simulink model "Aufiero_slew_pointing"  (R2021a)
settings: Solver=VariableStepAuto  StartTime=0.0  StopTime=100  RelTol=1e-3
settings Model: Creator=691615  LastModifiedBy=aufie
settings SolverCC: ZeroCrossAlgorithm=Adaptive  AlgebraicLoopSolver=TrustRegion
settings DebuggingCC: IgnoredZcDiagnostic=none  SFMachineParentedDataDiag=warning

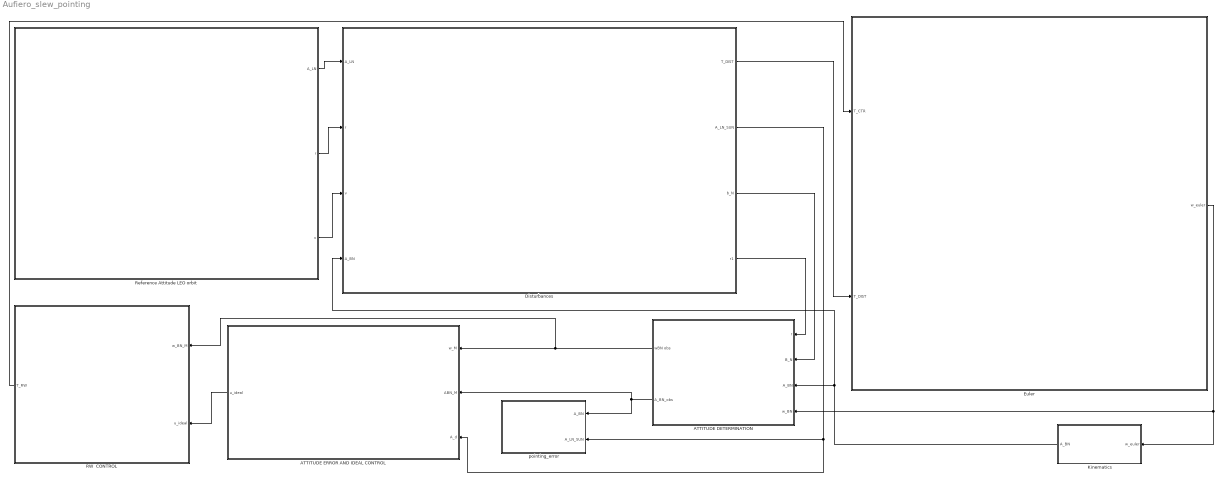
== system Aufiero_slew_pointing ==
  ATTITUDE DETERMINATION : Subsystem
  ATTITUDE ERROR AND IDEAL CONTROL : Subsystem
  Disturbances : Subsystem
  Euler : Subsystem
  Kinematics : Subsystem
  RW  CONTROL : Subsystem
  Reference Attitude LEO orbit : Subsystem
  pointing_error : Subsystem
  wires:
  ATTITUDE ERROR AND IDEAL CONTROL/1(u_ideal) -> RW  CONTROL/2(u_ideal)
  Kinematics/1(A_BN) -> ATTITUDE DETERMINATION/3(A_BN), Disturbances/4(A_BN)
  ATTITUDE DETERMINATION/2(A_BN_obs) -> ATTITUDE ERROR AND IDEAL CONTROL/2(ABN_M), pointing_error/1(A_BN)
  ATTITUDE DETERMINATION/1(wBN obs) -> ATTITUDE ERROR AND IDEAL CONTROL/1(w_M), RW  CONTROL/1(w_BN_M)
  Euler/1(w_euler) -> Kinematics/1(w_euler), ATTITUDE DETERMINATION/4(w_BN)
  RW  CONTROL/1(T_RW) -> Euler/1(T_CTR)
  Reference Attitude LEO orbit/3(v) -> Disturbances/3(v)
  Reference Attitude LEO orbit/1(A_LN) -> Disturbances/1(A_LN)
  Reference Attitude LEO orbit/2(r) -> Disturbances/2(r)
  Disturbances/1(T_DIST) -> Euler/2(T_DIST)
  Disturbances/2(A_LN_SUN) -> ATTITUDE ERROR AND IDEAL CONTROL/3(A_d), pointing_error/2(A_LN_SUN)
  Disturbances/4(r1) -> ATTITUDE DETERMINATION/1(r)
  Disturbances/3(b_N) -> ATTITUDE DETERMINATION/2(B_N)

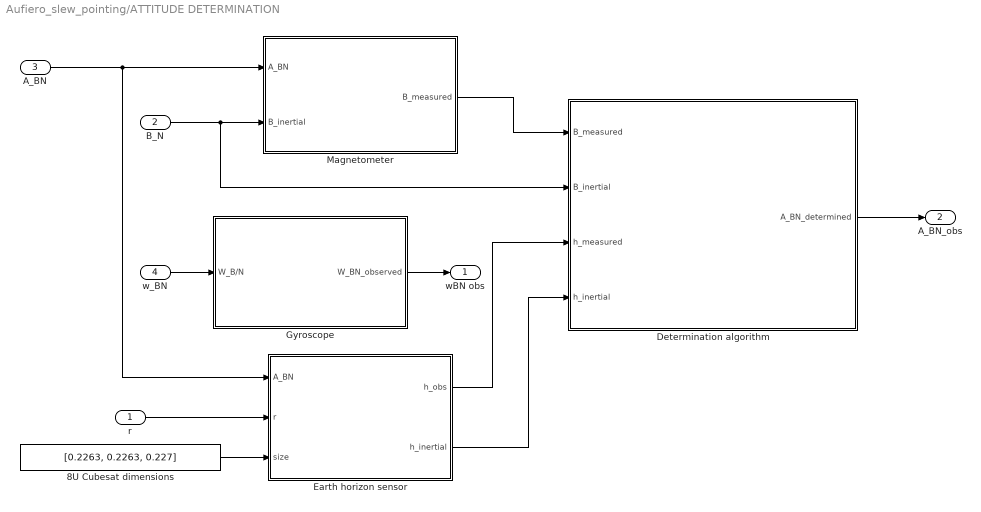
== system Aufiero_slew_pointing/ATTITUDE DETERMINATION ==
  r : Inport
  B_N : Inport  Port=2
  A_BN : Inport  Port=3
  w_BN : Inport  Port=4
  8U Cubesat dimensions : Constant  Value=[0.2263, 0.2263, 0.227]
  "Determination algorithm " : Subsystem
  Earth horizon sensor : Subsystem
  Gyroscope : Subsystem
  Magnetometer : Subsystem
  wBN obs : Outport  VectorParamsAs1DForOutWhenUnconnected=off
  A_BN_obs : Outport  Port=2  VectorParamsAs1DForOutWhenUnconnected=off
  wires:
  Earth horizon sensor/2(h_inertial) -> "Determination algorithm "/4(h_inertial)
  B_N/1 -> "Determination algorithm "/2(B_inertial), Magnetometer/2(B_inertial)
  w_BN/1 -> Gyroscope/1(W_B/N)
  "Determination algorithm "/1(A_BN_determined) -> A_BN_obs/1
  A_BN/1 -> Earth horizon sensor/1(A_BN), Magnetometer/1(A_BN)
  Earth horizon sensor/1(h_obs) -> "Determination algorithm "/3(h_measured)
  r/1 -> Earth horizon sensor/2(r)
  Gyroscope/1(W_BN_observed) -> wBN obs/1
  Magnetometer/1(B_measured) -> "Determination algorithm "/1(B_measured)
  8U Cubesat dimensions/1 -> Earth horizon sensor/3(size)

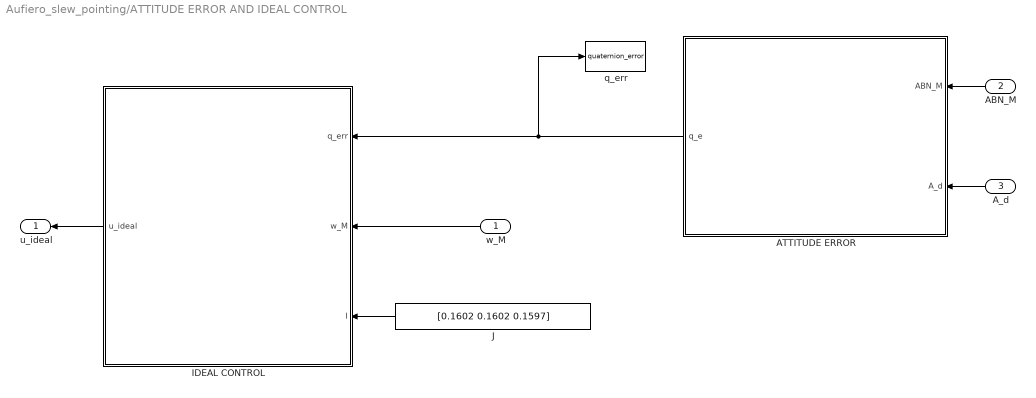
== system Aufiero_slew_pointing/ATTITUDE ERROR AND IDEAL CONTROL ==
  w_M : Inport
  ABN_M : Inport  Port=2
  A_d : Inport  Port=3
  ATTITUDE ERROR : MATLAB Function  TreatAsAtomicUnit=on
  IDEAL CONTROL : MATLAB Function  TreatAsAtomicUnit=on
  J : Constant  Value=[0.1602 0.1602 0.1597]
  q_err : ToWorkspace  VariableName=quaternion_error  SaveFormat=Timeseries  SampleTime=-1
  u_ideal : Outport  VectorParamsAs1DForOutWhenUnconnected=off
  wires:
  J/1 -> IDEAL CONTROL/3(I)
  w_M/1 -> IDEAL CONTROL/2(w_M)
  ABN_M/1 -> ATTITUDE ERROR/1(ABN_M)
  IDEAL CONTROL/1(u_ideal) -> u_ideal/1
  ATTITUDE ERROR/1(q_e) -> q_err/1, IDEAL CONTROL/1(q_err)
  A_d/1 -> ATTITUDE ERROR/2(A_d)

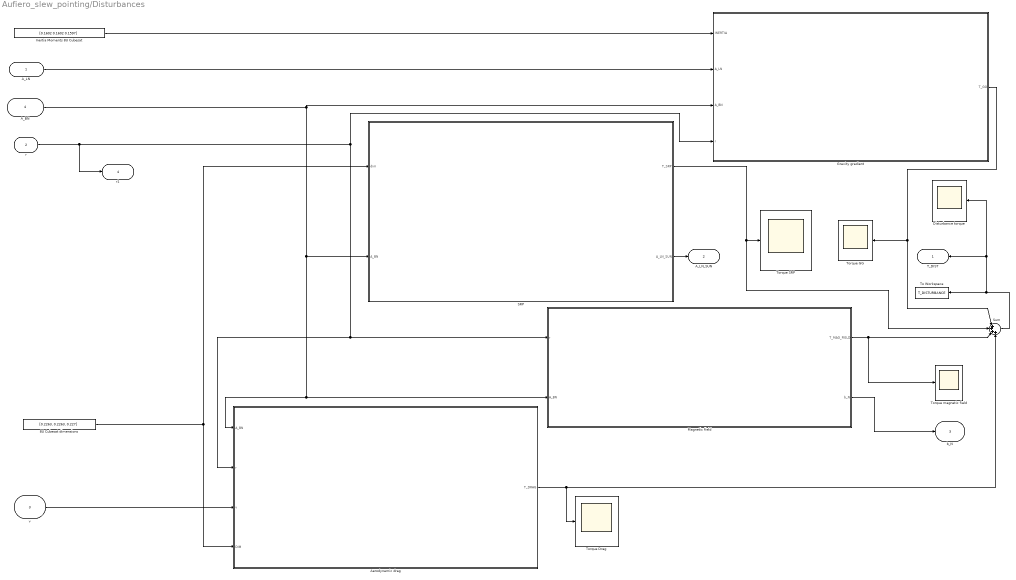
== system Aufiero_slew_pointing/Disturbances ==
  A_LN : Inport
  r : Inport  Port=2
  v : Inport  Port=3
  A_BN : Inport  Port=4
  8U Cubesat dimensions : Constant  Value=[0.2263, 0.2263, 0.227]
  Aerodynamic drag : Subsystem
  Disturbance torque : Scope
  Gravity gradient : Subsystem
  Inertia Moments 8U Cubesat : Constant  Value=[0.1602 0.1602 0.1597]
  Magnetic field : Subsystem
  SRP : Subsystem
  Sum : Sum  Inputs=|++++
  To Workspace : ToWorkspace  VariableName=T_DISTURBANCE  SaveFormat=Timeseries  SampleTime=-1
  Torque Drag : Scope
  Torque GG : Scope
  Torque SRP : Scope
  Torque magnetic field : Scope
  T_DIST : Outport  VectorParamsAs1DForOutWhenUnconnected=off
  A_LN_SUN : Outport  Port=2  VectorParamsAs1DForOutWhenUnconnected=off
  b_N : Outport  Port=3  VectorParamsAs1DForOutWhenUnconnected=off
  r1 : Outport  Port=4  VectorParamsAs1DForOutWhenUnconnected=off
  wires:
  r/1 -> Gravity gradient/4(r), Aerodynamic drag/2(r), Magnetic field/1(r), r1/1
  v/1 -> Aerodynamic drag/3(v)
  8U Cubesat dimensions/1 -> SRP/1(dim), Aerodynamic drag/4(DIM)
  Inertia Moments 8U Cubesat/1 -> Gravity gradient/1(INERTIA)
  A_LN/1 -> Gravity gradient/2(A_LN)
  Gravity gradient/1(T_GG) -> Torque GG/1, Sum/1
  SRP/1(T_SRP) -> Sum/2, Torque SRP/1
  Aerodynamic drag/1(T_DRAG) -> Sum/4, Torque Drag/1
  Magnetic field/1(T_MAG_FIELD) -> Torque magnetic field/1, Sum/3
  Magnetic field/2(b_N) -> b_N/1
  A_BN/1 -> Gravity gradient/3(A_BN), SRP/2(A_BN), Aerodynamic drag/1(A_BN), Magnetic field/2(A_BN)
  Sum/1 -> Disturbance torque/1, T_DIST/1, To Workspace/1
  SRP/2(A_LN_SUN) -> A_LN_SUN/1

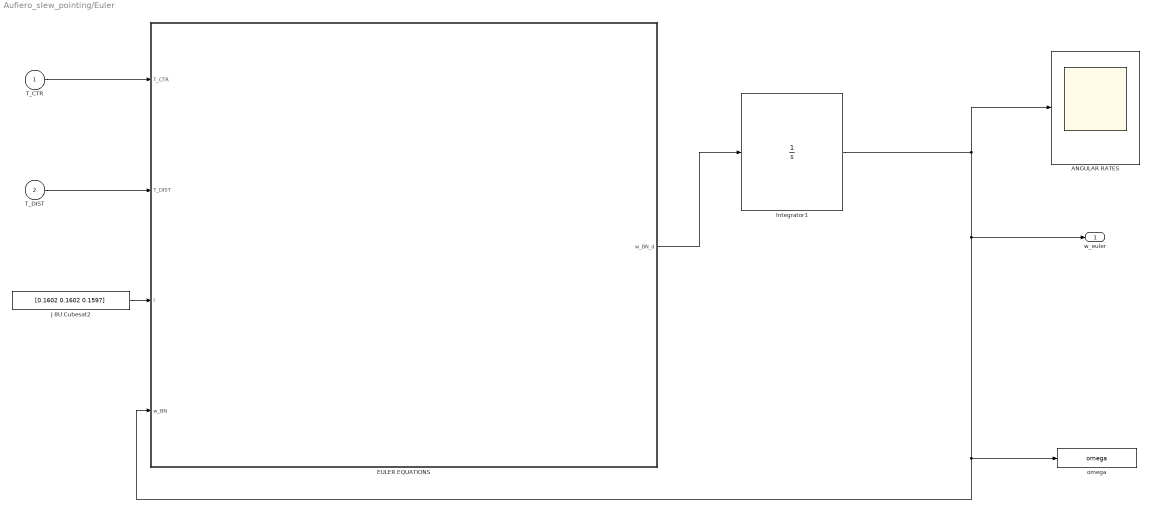
== system Aufiero_slew_pointing/Euler ==
  T_CTR : Inport
  T_DIST : Inport  Port=2
  ANGULAR RATES : Scope
  EULER EQUATIONS : MATLAB Function  TreatAsAtomicUnit=on
  Integrator1 : Integrator  InitialCondition=[0 0 0]
  J 8U Cubesat2 : Constant  Value=[0.1602 0.1602 0.1597]
  omega : ToWorkspace  VariableName=omega  SaveFormat=Timeseries  SampleTime=-1
  w_euler : Outport  VectorParamsAs1DForOutWhenUnconnected=off
  wires:
  T_CTR/1 -> EULER EQUATIONS/1(T_CTR)
  EULER EQUATIONS/1(w_BN_d) -> Integrator1/1
  T_DIST/1 -> EULER EQUATIONS/2(T_DIST)
  Integrator1/1 -> ANGULAR RATES/1, w_euler/1, EULER EQUATIONS/4(w_BN), omega/1
  J 8U Cubesat2/1 -> EULER EQUATIONS/3(I)

== system Aufiero_slew_pointing/Kinematics ==
  w_euler : Inport
  Attitude matrix quaternions : MATLAB Function  TreatAsAtomicUnit=on
  Integrator2 : Integrator  InitialCondition=[0 0 0 1]
  "Orthonorm. quaternions " : MATLAB Function  TreatAsAtomicUnit=on
  "Quaternions kinematics " : MATLAB Function  TreatAsAtomicUnit=on
  A_BN : Outport  VectorParamsAs1DForOutWhenUnconnected=off
  wires:
  w_euler/1 -> "Quaternions kinematics "/1(w)
  "Orthonorm. quaternions "/1(q_ortho) -> Attitude matrix quaternions/1(q), "Quaternions kinematics "/2(q)
  "Quaternions kinematics "/1(q_dot) -> Integrator2/1
  Integrator2/1 -> "Orthonorm. quaternions "/1(q)
  Attitude matrix quaternions/1(A_BN) -> A_BN/1

== system Aufiero_slew_pointing/RW  CONTROL ==
  w_BN_M : Inport
  u_ideal : Inport  Port=2
  RW REAL CONTROL : Subsystem
  TORQUE RW : Scope
  To Workspace : ToWorkspace  VariableName=T_RW  SaveFormat=Timeseries  SampleTime=-1
  T_RW : Outport  VectorParamsAs1DForOutWhenUnconnected=off
  wires:
  w_BN_M/1 -> RW REAL CONTROL/1(w_BN_obs)
  RW REAL CONTROL/1(T_RW) -> To Workspace/1, TORQUE RW/1, T_RW/1
  u_ideal/1 -> RW REAL CONTROL/2(u_ideal)

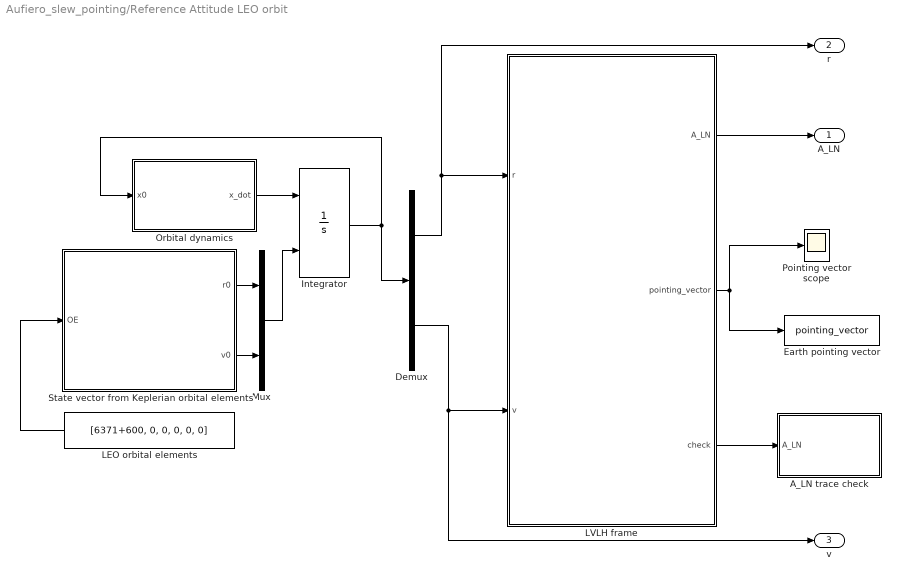
== system Aufiero_slew_pointing/Reference Attitude LEO orbit ==
  A_LN trace check : Subsystem
  Demux : Demux  Outputs=2
  Earth pointing vector : ToWorkspace  VariableName=pointing_vector  SampleTime=-1
  Integrator : Integrator  InitialConditionSource=external
  "LEO orbital elements " : Constant  Value=[6371+600, 0, 0, 0, 0, 0]
  LVLH frame : MATLAB Function  TreatAsAtomicUnit=on
  Mux : Mux  Inputs=2
  Orbital dynamics : MATLAB Function  TreatAsAtomicUnit=on
  Pointing vector scope : Scope
  State vector from Keplerian orbital elements : MATLAB Function  TreatAsAtomicUnit=on
  A_LN : Outport  VectorParamsAs1DForOutWhenUnconnected=off
  r : Outport  Port=2  VectorParamsAs1DForOutWhenUnconnected=off
  v : Outport  Port=3  VectorParamsAs1DForOutWhenUnconnected=off
  wires:
  Integrator/1 -> Demux/1, Orbital dynamics/1(x0)
  State vector from Keplerian orbital elements/2(v0) -> Mux/2
  Demux/2 -> v/1, LVLH frame/2(v)
  Demux/1 -> r/1, LVLH frame/1(r)
  Mux/1 -> Integrator/2
  Orbital dynamics/1(x_dot) -> Integrator/1
  State vector from Keplerian orbital elements/1(r0) -> Mux/1
  "LEO orbital elements "/1 -> State vector from Keplerian orbital elements/1(OE)
  LVLH frame/2(pointing_vector) -> Pointing vector scope/1, Earth pointing vector/1
  LVLH frame/3(check) -> A_LN trace check/1(A_LN)
  LVLH frame/1(A_LN) -> A_LN/1

== system Aufiero_slew_pointing/pointing_error ==
  A_BN : Inport
  A_LN_SUN : Inport  Port=2
  " Pointing Angle Accuracy" : MATLAB Function  TreatAsAtomicUnit=on
  pointing_err : Scope
  q_err2 : ToWorkspace  VariableName=pointing_err  SampleTime=-1
  wires:
  A_BN/1 -> " Pointing Angle Accuracy"/1(A_BN)
  " Pointing Angle Accuracy"/1(alfa_pointing_deg) -> pointing_err/1, q_err2/1
  A_LN_SUN/1 -> " Pointing Angle Accuracy"/2(A_LN)

== system Aufiero_slew_pointing/ATTITUDE DETERMINATION/Determination algorithm  ==
  B_measured : Inport
  B_inertial : Inport  Port=2
  h_measured : Inport  Port=3
  h_inertial : Inport  Port=4
  Static determination : Subsystem
  A_BN_determined : Outport  VectorParamsAs1DForOutWhenUnconnected=off
  wires:
  h_inertial/1 -> Static determination/1(h_inertial)
  h_measured/1 -> Static determination/2(h_measured)
  B_measured/1 -> Static determination/4(B_measured)
  Static determination/1(A_BN_determined) -> A_BN_determined/1
  B_inertial/1 -> Static determination/3(B_inertial)

== system Aufiero_slew_pointing/ATTITUDE DETERMINATION/Earth horizon sensor ==
  A_BN : Inport
  r : Inport  Port=2
  size : Inport  Port=3
  Earth Horizon sensor : MATLAB Function  TreatAsAtomicUnit=on
  h_obs : Outport  VectorParamsAs1DForOutWhenUnconnected=off
  h_inertial : Outport  Port=2  VectorParamsAs1DForOutWhenUnconnected=off
  wires:
  r/1 -> Earth Horizon sensor/2(r)
  size/1 -> Earth Horizon sensor/3(size)
  Earth Horizon sensor/1(h_obs) -> h_obs/1
  Earth Horizon sensor/2(h_body) -> h_inertial/1
  A_BN/1 -> Earth Horizon sensor/1(A_BN)

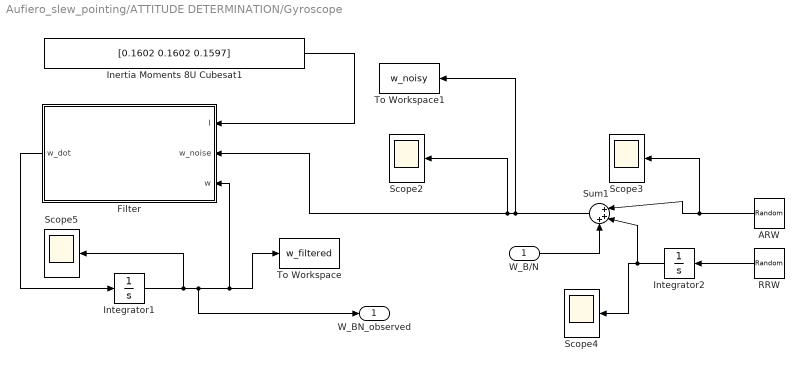
== system Aufiero_slew_pointing/ATTITUDE DETERMINATION/Gyroscope ==
  W_B/N : Inport
  ARW : RandomNumber  Variance=(0.15*pi/180/3600)*sqrt(1/262)  SampleTime=1/262
  "Filter " : MATLAB Function  TreatAsAtomicUnit=on
  Inertia Moments 8U Cubesat1 : Constant  Value=[0.1602 0.1602 0.1597]
  Integrator1 : Integrator  InitialCondition=[0.1 0.1 0.1]
  Integrator2 : Integrator
  RRW : RandomNumber  Variance=(0.3*pi/180/3600)*sqrt(1/262)  SampleTime=1/262
  Scope{2..5} (4 alike) : Scope
  Sum1 : Sum  Inputs=|+++
  To Workspace : ToWorkspace  VariableName=w_filtered  SaveFormat=Timeseries  SampleTime=-1
  To Workspace1 : ToWorkspace  VariableName=w_noisy  SaveFormat=Timeseries  SampleTime=-1
  W_BN_observed : Outport  VectorParamsAs1DForOutWhenUnconnected=off
  wires:
  "Filter "/1(w_dot) -> Integrator1/1
  W_B/N/1 -> Sum1/3
  Sum1/1 -> "Filter "/2(w_noise), Scope2/1, To Workspace1/1
  Integrator2/1 -> Scope4/1, Sum1/2
  Inertia Moments 8U Cubesat1/1 -> "Filter "/1(I)
  Integrator1/1 -> W_BN_observed/1, "Filter "/3(w), To Workspace/1, Scope5/1
  RRW/1 -> Integrator2/1
  ARW/1 -> Scope3/1, Sum1/1

== system Aufiero_slew_pointing/ATTITUDE DETERMINATION/Magnetometer ==
  A_BN : Inport
  B_inertial : Inport  Port=2
  MATLAB Function5 : MATLAB Function  TreatAsAtomicUnit=on
  B_measured : Outport  VectorParamsAs1DForOutWhenUnconnected=off
  wires:
  MATLAB Function5/1(b_B) -> B_measured/1
  B_inertial/1 -> MATLAB Function5/1(b_N)
  A_BN/1 -> MATLAB Function5/2(A_BN)

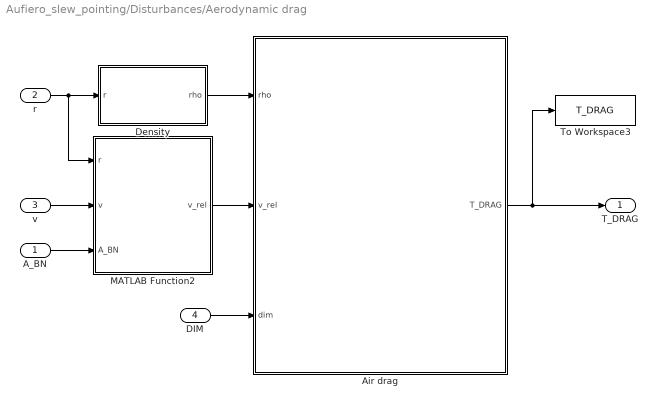
== system Aufiero_slew_pointing/Disturbances/Aerodynamic drag ==
  A_BN : Inport
  r : Inport  Port=2
  v : Inport  Port=3
  DIM : Inport  Port=4
  Air drag : MATLAB Function  TreatAsAtomicUnit=on
  Density : MATLAB Function  TreatAsAtomicUnit=on
  MATLAB Function2 : MATLAB Function  TreatAsAtomicUnit=on
  To Workspace3 : ToWorkspace  VariableName=T_DRAG  SaveFormat=Timeseries  SampleTime=-1
  T_DRAG : Outport  VectorParamsAs1DForOutWhenUnconnected=off
  wires:
  MATLAB Function2/1(v_rel) -> Air drag/2(v_rel)
  A_BN/1 -> MATLAB Function2/3(A_BN)
  Density/1(rho) -> Air drag/1(rho)
  v/1 -> MATLAB Function2/2(v)
  r/1 -> MATLAB Function2/1(r), Density/1(r)
  DIM/1 -> Air drag/3(dim)
  Air drag/1(T_DRAG) -> T_DRAG/1, To Workspace3/1

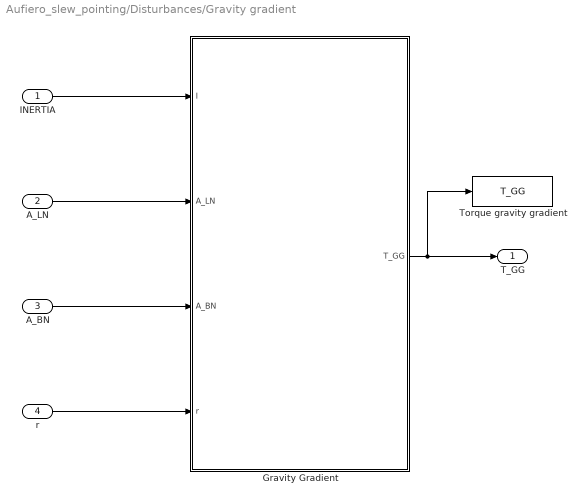
== system Aufiero_slew_pointing/Disturbances/Gravity gradient ==
  INERTIA : Inport
  A_LN : Inport  Port=2
  A_BN : Inport  Port=3
  r : Inport  Port=4
  Gravity Gradient : MATLAB Function  TreatAsAtomicUnit=on
  Torque gravity gradient : ToWorkspace  VariableName=T_GG  SaveFormat=Timeseries  SampleTime=-1
  T_GG : Outport  VectorParamsAs1DForOutWhenUnconnected=off
  wires:
  Gravity Gradient/1(T_GG) -> T_GG/1, Torque gravity gradient/1
  INERTIA/1 -> Gravity Gradient/1(I)
  A_LN/1 -> Gravity Gradient/2(A_LN)
  A_BN/1 -> Gravity Gradient/3(A_BN)
  r/1 -> Gravity Gradient/4(r)

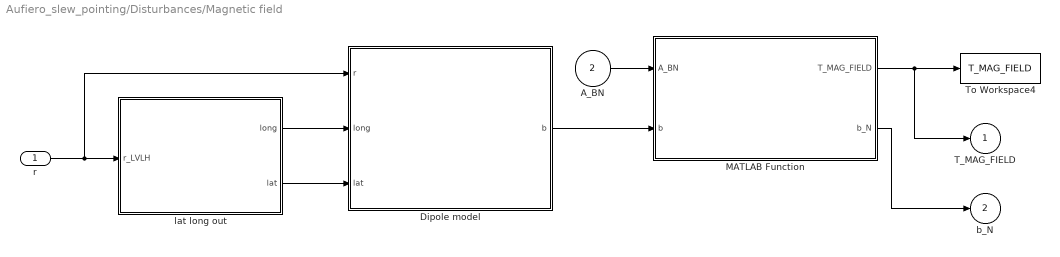
== system Aufiero_slew_pointing/Disturbances/Magnetic field ==
  r : Inport
  A_BN : Inport  Port=2
  Dipole model : MATLAB Function  TreatAsAtomicUnit=on
  MATLAB Function : MATLAB Function  TreatAsAtomicUnit=on
  To Workspace4 : ToWorkspace  VariableName=T_MAG_FIELD  SaveFormat=Timeseries  SampleTime=-1
  "lat long out " : MATLAB Function  TreatAsAtomicUnit=on
  T_MAG_FIELD : Outport  VectorParamsAs1DForOutWhenUnconnected=off
  b_N : Outport  Port=2  VectorParamsAs1DForOutWhenUnconnected=off
  wires:
  r/1 -> "lat long out "/1(r_LVLH), Dipole model/1(r)
  A_BN/1 -> MATLAB Function/1(A_BN)
  Dipole model/1(b) -> MATLAB Function/2(b)
  MATLAB Function/1(T_MAG_FIELD) -> T_MAG_FIELD/1, To Workspace4/1
  MATLAB Function/2(b_N) -> b_N/1
  "lat long out "/1(long) -> Dipole model/2(long)
  "lat long out "/2(lat) -> Dipole model/3(lat)

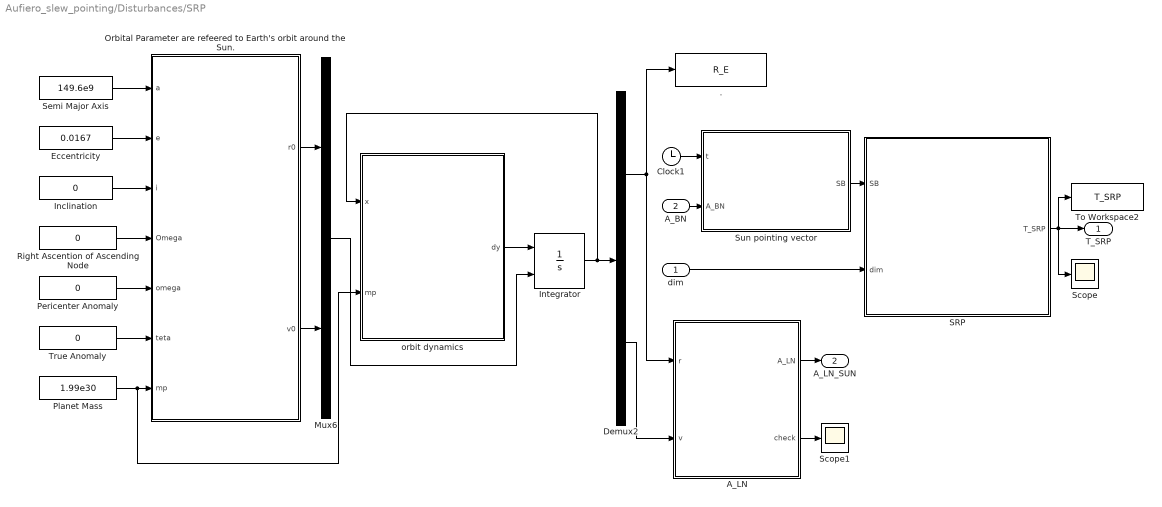
== system Aufiero_slew_pointing/Disturbances/SRP ==
  dim : Inport
  A_BN : Inport  Port=2
  . : ToWorkspace  VariableName=R_E  SampleTime=-1
      settings: Save2DSignal=2-D array (concatenate along first dimension)
  A_LN : MATLAB Function  TreatAsAtomicUnit=on
  Clock1 : Clock
  Demux2 : Demux  Outputs=2
  Eccentricity : Constant  Value=0.0167
  Inclination : Constant  Value=0
  Integrator : Integrator  InitialConditionSource=external
  Mux6 : Mux  Inputs=2
  "Orbital Parameter are refeered to Earth's orbit around the Sun.   " : MATLAB Function  TreatAsAtomicUnit=on
  Pericenter Anomaly : Constant  Value=0
  Planet Mass : Constant  Value=1.99e30
  Right Ascention of Ascending Node : Constant  Value=0
  SRP : MATLAB Function  TreatAsAtomicUnit=on
  Scope : Scope
  Scope1 : Scope
  Semi Major Axis : Constant  Value=149.6e9
  Sun pointing vector : MATLAB Function  TreatAsAtomicUnit=on
  To Workspace2 : ToWorkspace  VariableName=T_SRP  SaveFormat=Timeseries  SampleTime=-1
  True Anomaly : Constant  Value=0
  orbit dynamics : MATLAB Function  TreatAsAtomicUnit=on
  T_SRP : Outport  VectorParamsAs1DForOutWhenUnconnected=off
  A_LN_SUN : Outport  Port=2
  wires:
  Integrator/1 -> Demux2/1, orbit dynamics/1(x)
  Right Ascention of Ascending Node/1 -> "Orbital Parameter are refeered to Earth's orbit around the Sun.   "/4(Omega)
  A_LN/1(A_LN) -> A_LN_SUN/1
  A_LN/2(check) -> Scope1/1
  "Orbital Parameter are refeered to Earth's orbit around the Sun.   "/2(v0) -> Mux6/2
  Planet Mass/1 -> orbit dynamics/2(mp), "Orbital Parameter are refeered to Earth's orbit around the Sun.   "/7(mp)
  Demux2/2 -> A_LN/2(v)
  SRP/1(T_SRP) -> To Workspace2/1, T_SRP/1, Scope/1
  Demux2/1 -> ./1, A_LN/1(r)
  Eccentricity/1 -> "Orbital Parameter are refeered to Earth's orbit around the Sun.   "/2(e)
  Semi Major Axis/1 -> "Orbital Parameter are refeered to Earth's orbit around the Sun.   "/1(a)
  Inclination/1 -> "Orbital Parameter are refeered to Earth's orbit around the Sun.   "/3(i)
  Pericenter Anomaly/1 -> "Orbital Parameter are refeered to Earth's orbit around the Sun.   "/5(omega)
  Mux6/1 -> Integrator/2
  "Orbital Parameter are refeered to Earth's orbit around the Sun.   "/1(r0) -> Mux6/1
  orbit dynamics/1(dy) -> Integrator/1
  True Anomaly/1 -> "Orbital Parameter are refeered to Earth's orbit around the Sun.   "/6(teta)
  dim/1 -> SRP/2(dim)
  Clock1/1 -> Sun pointing vector/1(t)
  A_BN/1 -> Sun pointing vector/2(A_BN)
  Sun pointing vector/1(SB) -> SRP/1(SB)

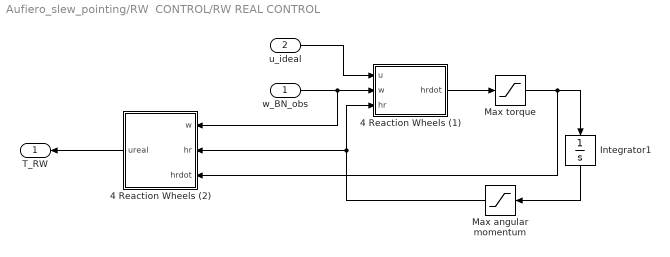
== system Aufiero_slew_pointing/RW  CONTROL/RW REAL CONTROL ==
  w_BN_obs : Inport
  u_ideal : Inport  Port=2
  4 Reaction Wheels (1) : MATLAB Function  TreatAsAtomicUnit=on
  4 Reaction Wheels (2) : MATLAB Function  TreatAsAtomicUnit=on
  Integrator1 : Integrator  InitialCondition=[0 0 0 0]
  Max angular momentum : Saturate  UpperLimit=0.34  LowerLimit=-0.34
  Max torque : Saturate  UpperLimit=0.015  LowerLimit=-0.015
  T_RW : Outport  VectorParamsAs1DForOutWhenUnconnected=off
  wires:
  Max torque/1 -> 4 Reaction Wheels (2)/3(hrdot), Integrator1/1
  Integrator1/1 -> Max angular momentum/1
  4 Reaction Wheels (1)/1(hrdot) -> Max torque/1
  Max angular momentum/1 -> 4 Reaction Wheels (1)/3(hr), 4 Reaction Wheels (2)/2(hr)
  w_BN_obs/1 -> 4 Reaction Wheels (2)/1(w), 4 Reaction Wheels (1)/2(w)
  u_ideal/1 -> 4 Reaction Wheels (1)/1(u)
  4 Reaction Wheels (2)/1(ureal) -> T_RW/1

== system Aufiero_slew_pointing/Reference Attitude LEO orbit/A_LN trace check ==
  A_LN : Inport
  Orthonormality check : MATLAB Function  TreatAsAtomicUnit=on
  Trace A_LN : ToWorkspace  VariableName=A_LN_trace  SaveFormat=Timeseries  SampleTime=-1
  Trace A_LN scope : Scope
  wires:
  A_LN/1 -> Orthonormality check/1(A_LN)
  Orthonormality check/1(t) -> Trace A_LN scope/1, Trace A_LN/1

== system Aufiero_slew_pointing/ATTITUDE DETERMINATION/Determination algorithm /Static determination ==
  h_inertial : Inport
  h_measured : Inport  Port=2
  B_inertial : Inport  Port=3
  B_measured : Inport  Port=4
  attitude determination : MATLAB Function  TreatAsAtomicUnit=on
  A_BN_determined : Outport  VectorParamsAs1DForOutWhenUnconnected=off
  wires:
  B_inertial/1 -> attitude determination/3(B_inertial)
  h_measured/1 -> attitude determination/2(h_measured)
  attitude determination/1(A_B_N) -> A_BN_determined/1
  h_inertial/1 -> attitude determination/1(h_inertial)
  B_measured/1 -> attitude determination/4(B_measured)

== matlab function Aufiero_slew_pointing/Disturbances/Aerodynamic drag/Air drag ==
  data: rho input; T_DRAG output; v_rel input; dim input
function T_DRAG = drag(rho,v_rel,dim)

air_dragT  = zeros(3,6);
air_dragF  = zeros(3,6);
cos_theta  = zeros(1,6);
T_DRAG = zeros(3,1); 

Cd = 2.2;

    % Normal to surfaces
    n = zeros(3,6);
    n(:,1) = [ 1  0  0 ]';
    n(:,2) = [ 0  1  0 ]';
    n(:,3) = [ 0  0  1 ]';
    n(:,4) = [-1  0  0 ]';
    n(:,5) = [ 0 -1  0 ]';
    n(:,6) = [ 0  0 -1 ]';
  
    b = zeros (3,6); % Offset mass centre - pressure centre
    b(:,1) = 0.1.*[    0    dim(2)  dim(3)]';
    b(:,2) = 0.1.*[ dim(1)     0    dim(3)]';
    b(:,3) = 0.1.*[ dim(1)   dim(2)    0  ]';
    b(:,4) = 0.1.*[    0    dim(2)  dim(3)]';
    b(:,5) = 0.1.*[ dim(1)     0    dim(3)]';
    b(:,6) = 0.1.*[ dim(1)   dim(2)    0  ]';
    
    % Area of surfaces
    A = zeros (6,1);
    A(1) = dim(3) * dim(2);
    A(4) = dim(3) * dim(2);
    A(2) = dim(3) * dim(1);
    A(5) = dim(3) * dim(1);
    A(3) = dim(2) * dim(1);
    A(6) = dim(2) * dim(1);
    
    
    
    for i = 1:6
        
        cos_theta(i) = dot(n(:,i),v_rel/norm(v_rel));
        
        if        cos_theta(i) < 0
                  air_dragT(:,i) = 0;
                  
                  
        
        else     
                
                  air_dragF = -0.5*rho*Cd*(norm(v_rel))^2*v_rel/norm(v_rel)*cos_theta(i)*A(i);
        
                  air_dragT(:,i) = cross(b(:,i),air_dragF);
                  
        end
        
    end
    
    T_DRAG = air_dragT(:,1) + air_dragT(:,2) + air_dragT(:,3) + air_dragT(:,4) + air_dragT(:,5) + air_dragT(:,6);
                 
                 
end

== matlab function Aufiero_slew_pointing/Disturbances/Aerodynamic drag/Density ==
  data: r input; rho output
function rho = exp_density_model(r)

r = norm(r);
h = (r - 6371000)*10^-3; % actual height [km]

if          h>=0 && h<25
            h_0 =   0; rho_0 =  1.225    ; H =   7.249;
    
elseif      h>=25 && h<30
            h_0 =   25; rho_0 = 3.899e-2 ; H =   6.349;
            
elseif      h>=30 && h<40
            h_0 =   30; rho_0 = 1.774e-2 ; H =   6.682;
                       
elseif      h>=40 && h<50
            h_0 =   40; rho_0 = 3.972e-3 ; H =   7.554;
            
elseif      h>=50 && h<60
            h_0 =   50; rho_0 = 1.057e-3 ; H =   8.382;
            
elseif      h>=60 && h<70
            h_0 =   60; rho_0 = 3.206e-4 ; H =   7.714;
            
elseif      h>=70 && h<80
            h_0 =   70; rho_0 = 8.770e-5 ; H =   6.549;

elseif      h>=80 && h<90
            h_0 =   80; rho_0 = 1.905e-5 ; H =   5.799;
            
elseif      h>=90 && h<100
            h_0 =   90; rho_0 = 3.396e-6 ; H =   5.382;
            
elseif      h>=100 && h<110
            h_0 =  100; rho_0 = 5.297e-7 ; H =   5.877;            
            
elseif      h>=110 && h<120
            h_0 =  110; rho_0 = 9.661e-8 ; H =   7.263;
            
elseif      h>=120 && h<130
            h_0 =  120; rho_0 = 2.438e-8 ; H =   9.473;           
            
elseif      h>=130 && h<140
            h_0 =  130; rho_0 = 8.484e-9 ; H =  12.636;
            
elseif      h>=140 && h<150
            h_0 =  140; rho_0 = 3.845e-9 ; H =  16.149;            
            
elseif      h>=150 && h<180
            h_0 =  150; rho_0 = 2.070e-9 ; H =  22.523;            
            
elseif      h>=180 && h<200
            h_0 =  180; rho_0 = 5.464e-10; H =  29.740;
            
elseif      h>=200 && h<250
            h_0 =  200; rho_0 = 2.789e-10; H =  37.105;            
            
elseif      h>=250 && h<300
            h_0 =  250; rho_0 = 7.248e-11; H =  45.546;            
            
elseif      h>=300 && h<350
            h_0 =  300; rho_0 = 2.418e-11; H =  53.628;
            
elseif      h>=350 && h<400
            h_0 =  350; rho_0 = 9.158e-12; H =  53.298;            
            
elseif      h>=400 && h<450
            h_0 =  400; rho_0 = 3.725e-12; H =  58.515;
            
elseif      h>=450 && h<500
            h_0 =  450; rho_0 = 1.585e-12; H =  60.828;
            
elseif      h>=500 && h<600
            h_0 =  500; rho_0 = 6.967e-13; H =  63.822;
            
elseif      h>=600 && h<700
            h_0 =  600; rho_0 = 1.454e-13; H =  71.835;            
            
elseif      h>=700 && h<800
            h_0 =  700; rho_0 = 3.614e-14; H =  88.667;            
            
elseif      h>=800 && h<900
            h_0 =  800; rho_0 = 1.170e-14; H = 124.64;
            
elseif      h>=900 && h<1000
            h_0 =  900; rho_0 = 5.245e-15; H = 181.05;                       
         
else      
            h_0 = 1000; rho_0 = 3.019e-15; H = 268.00;
            
end


rho = rho_0*exp(-(h-h_0)/H);

== matlab function Aufiero_slew_pointing/Disturbances/Aerodynamic drag/MATLAB Function2 ==
  data: r input; v_rel output; v input; A_BN input
function v_rel = relative_velocity(r,v,A_BN)

 % relative velocity between air and spacecraft
 
 v_rel = zeros (3,1);
 
 
 v_rel(1) = v(1) + 0.000072921*r(2);
 v_rel(2) = v(2) - 0.000072921*r(1);
 v_rel(3) = v(3);
 
 v_rel = A_BN * v_rel;
 
end

== matlab function Aufiero_slew_pointing/ATTITUDE DETERMINATION/Magnetometer/MATLAB Function5 ==
  data: b_N input; A_BN input; b_B output
function b_B = magnetometer(b_N, A_BN)

% angle errors; should be 3, for simplicity here they are assumed to be
% equal to 5 deg for each axis

                      
psi = 5*pi/180; %[rad] angular error
theta = 5*pi/180; %[rad] angular error
phi = 5*pi/180; %[rad] angular error

A_eps = [cos(psi)*cos(theta),  cos(psi)*sin(theta)*sin(phi)+sin(psi)*cos(phi), -cos(psi)*sin(theta)*cos(phi)+sin(psi)*sin(phi);
        -sin(psi)*cos(theta), -sin(psi)*sin(theta)*sin(phi)+cos(psi)*cos(phi),  sin(psi)*sin(theta)*cos(phi)+cos(psi)*sin(phi);
              sin(theta),                -cos(theta)*sin(phi),                              cos(theta)*cos(phi)];


% measured magnetic field vector in the body frame
          
b_B = A_eps * A_BN * b_N;

== matlab function Aufiero_slew_pointing/Euler/EULER EQUATIONS ==
  data: T_CTR input; T_DIST input; I input; w_BN input; w_BN_d output
function w_BN_d = euler (T_CTR, T_DIST, I, w_BN)

% EULER EQUATIONS INLCUDING DISTURBANCES AND CONTROL TORQUES

w_BN_d = zeros (1,3);

% DISTURBANCES + CONTROL TORQUE
w_BN_d(1) = (I(2)-I(3))/I(1)*w_BN(2)*w_BN(3) + T_DIST(1)/I(1) + T_CTR(1)/I(1);
w_BN_d(2) = (I(3)-I(1))/I(2)*w_BN(1)*w_BN(3) + T_DIST(2)/I(2) + T_CTR(2)/I(2);
w_BN_d(3) = (I(1)-I(2))/I(3)*w_BN(1)*w_BN(2) + T_DIST(3)/I(3) + T_CTR(3)/I(3);


w_BN_d = [w_BN_d(1) w_BN_d(2) w_BN_d(3)];


end

== matlab function Aufiero_slew_pointing/Kinematics/Attitude matrix quaternions ==
  data: q input; A_BN output
%function [A, ea_q] = quat_to_DCM(q)
function A_BN  = quat_to_DCM(q)

%% Elements of the A matrix as f(q)

A11 = q(1)^2 - q(2)^2 - q(3)^2 + q(4)^2;
A12 = 2*(q(1)*q(2) + q(3)*q(4));
A13 = 2*(q(1)*q(3) - q(2)*q(4));

A21 = 2*(q(1)*q(2) - q(3)*q(4));
A22 = -q(1)^2 + q(2)^2 - q(3)^2 + q(4)^2;
A23 = 2*(q(2)*q(3) + q(1)*q(4));

A31 = 2*(q(1)*q(3) + q(2)*q(4));
A32 = 2*(q(2)*q(3) - q(1)*q(4));
A33 = -q(1)^2 - q(2)^2 + q(3)^2 + q(4)^2;

A_BN = [ A11 A12 A13
      A21 A22 A23
      A31 A32 A33  ];

% %% New Euler Angles
% 
% phi = acosd(A(3,3));
% theta = -atand(A(3,1)/A(3,2));
% psi = atand(A(1,3)/A(2,3));
% 
% ea_q = [phi theta psi];

end

== matlab function Aufiero_slew_pointing/Disturbances/Magnetic field/Dipole model ==
  data: r input; long input; b output; lat input
function b = dipole_model(r, long, lat)

n_pole = [cos(80.37*pi/180)*cos(-72.62*pi/180);
          cos(80.37*pi/180)*sin(-72.62*pi/180);
                sin(80.37*pi/180)];
m_hat = -n_pole;

% Gaussian coefficients - IGRF 2015
g10 = -29442.0; %[nT]
g11 = -1501.0; %[nT]
h11 = 4797.1; %[nT]
H0 = sqrt(g10^2 + g11^2 + h11^2);
R_earth = 6371;

r_unit = [cos(lat*pi/180)*cos(long*pi/180);
    cos(lat*pi/180)*sin(long*pi/180);
    sin(lat*pi/180)];

b = (R_earth/norm(r))^3*H0*(3*dot(m_hat,r_unit)*r_unit - m_hat); %[nT]

end

== matlab function Aufiero_slew_pointing/Kinematics/Orthonorm. quaternions  ==
  data: q input; q_ortho output
function q_ortho = orho_quat(q)

Q1 = q(1)^2;
Q2 = q(2)^2;
Q3 = q(3)^2;
Q4 = q(4)^2;

Q = Q1 + Q2 + Q3 + Q4;

q_ortho = q/Q;

== matlab function Aufiero_slew_pointing/Kinematics/Quaternions kinematics  ==
  data: w input; q_dot output; q input
function q_dot = fcn(w, q)
% The input quaternions are already the orthonormalized ones

W = [   0   w(3)    -w(2)   w(1); 
      -w(3)  0       w(1)   w(2); 
       w(2) -w(1)     0     w(3); 
      -w(1) -w(2)   -w(3)    0   ];

q_dot = 0.5 * (W * q);

== matlab function Aufiero_slew_pointing/Disturbances/SRP/Sun pointing vector ==
  data: t input; SB output; A_BN input
function SB = sun_pointing(t, A_BN)

n = 2*pi/(365.25*3600*24); % Mean motion 
t0 = 150*n; % Initial time for the simulation (assuming 150s from previous detumbling)
eps = 23.45*pi/180; % Ecliptic inclination

% Sun pointing vector in inertial sun-centered reference frame
SN = [cos(n*t+t0); sin(n*t+t0)*cos(eps); sin(n*t+t0)*sin(eps)];

% Sun pointing vector in body frame
SB = A_BN * SN;

== matlab function Aufiero_slew_pointing/Disturbances/Magnetic field/lat long out  ==
  data: r_LVLH input; long output; lat output
function [long, lat] = ra_dec_from_r(r_LVLH)
% This function calculates the right ascension and the declination
% from the geocentric equatorial position vector.
%
% INPUT
%   r       position vector in ECI frame        [km]        [1x3]
%
% OUTPUT
%   ra      right ascension                     [deg]
%   dec     declination                         [deg]
%
%   Verified by Daniele Leuteri Costanzo

%% CALCULATE DIRECTION COSINES
l = r_LVLH(1)/norm(r_LVLH);
m = r_LVLH(2)/norm(r_LVLH);
n = r_LVLH(3)/norm(r_LVLH);

%% CALCULATE DECLINATION

lat = asind(n);

%% CALCULATE RIGHT ASCENSION

    if m > 0
        long = acosd(l/cosd(lat));
    else
        long = 360 - acosd(l/cosd(lat));
    end
end

== matlab function Aufiero_slew_pointing/Disturbances/Magnetic field/MATLAB Function ==
  data: A_BN input; T_MAG_FIELD output; b input; b_N output
function [T_MAG_FIELD, b_N] = magneticTorques(A_BN, b)

m_res = [0.1; 0.1; 0.1]; % residual magnetic induction

b_N = b*1e-9; %[T]

b_B = A_BN*b_N; %[T] magnetic field in the body frame

T_MAG_FIELD = cross(m_res,b_B); %[N.m]

end

== matlab function Aufiero_slew_pointing/ATTITUDE DETERMINATION/Earth horizon sensor/Earth Horizon sensor ==
  settings: updateMethod=DISCRETE
  data: A_BN input; h_obs output; r input; h_body output; size input
function [h_obs,h_body] = Earth_hor_sens(A_BN,r,size)

accuracy = 6*1/60;               % [deg]     6 arcminutes

psi = accuracy*pi/180;
phi = accuracy*pi/180;
theta = accuracy*pi/180;

A_eps = zeros(3,3);
A_eps(1,1) = cos(psi)*cos(phi);
A_eps(1,2) = cos(psi)*sin(theta)*sin(phi)+sin(psi)*cos(phi);
A_eps(1,3) = -cos(psi)*sin(theta)*cos(phi)+sin(psi)*sin(phi);
A_eps(2,1) = -sin(psi)*cos(phi);
A_eps(2,2) = -sin(psi)*sin(theta)*sin(phi)+cos(psi)*cos(phi);
A_eps(2,3) = sin(psi)*sin(theta)*cos(phi)+cos(psi)*sin(phi);
A_eps(3,1) = sin(theta);
A_eps(3,2) = -cos(theta)*sin(phi);
A_eps(3,3) = cos(theta)*cos(psi);

v_n = -r + [size(1)/2;0;0];

h_body = A_BN * v_n;

h_obs = A_eps*h_body;

== matlab function Aufiero_slew_pointing/ATTITUDE DETERMINATION/Gyroscope/Filter  ==
  data: I input; w_noise input; w input; w_dot output
function w_dot = filter_gyro(I,w_noise, w)

k1 = 0.08;
I_x = I(1);
I_y = I(2);
I_z = I(3);

w_dot=zeros(3,1);
w_dot(1) =  ((I_y-I_z)/I_x)*w(2)*w(3) + k1 * (w_noise(1)-w(1));
w_dot(2) =  ((I_z-I_x)/I_y)*w(1)*w(3) + k1 * (w_noise(2)-w(2));
w_dot(3) =  ((I_x-I_y)/I_z)*w(1)*w(2) + k1 * (w_noise(3)-w(3));

== matlab function Aufiero_slew_pointing/ATTITUDE ERROR AND IDEAL CONTROL/ATTITUDE ERROR ==
  data: ABN_M input; q_e output; A_d input
function q_e = attError(ABN_M,A_d)

% Attitude error in DCM form
A_e = ABN_M * A_d';

% Attitude error in quaternion form
q_e = dcm2q(A_e);



end

== matlab function Aufiero_slew_pointing/ATTITUDE ERROR AND IDEAL CONTROL/IDEAL CONTROL ==
  data: q_err input; u_ideal output; w_M input; I input
function u_ideal = idealCtr(q_err, w_M, I)


k1 = 0.185;
k2 = k1^2/2;
J = diag(I);

w_err = w_M - [0;0;0];

% Pointing control
% H(q4e) = 1 - q4e^2

u_ideal = cross (w_err, J*w_err) - k1 * w_err + k2 * (-q_err(4)) * q_err(1:3)';

% Slew control
% H(q4e) = 1 - q4e^2

%u_ideal = - k1 * w_err - k2 * (2*q_err(4)) * q_err(1:3)';



end

== matlab function Aufiero_slew_pointing/RW  CONTROL/RW REAL CONTROL/4 Reaction Wheels (1) ==
  data: u input; w input; hrdot output; hr input
function hrdot = RW1(u,w,hr)

A=[1 0 0 1/sqrt(3)
    0 1 0 1/sqrt(3)
    0 0 1 1/sqrt(3)];

Astar=pinv(A);

hrdot=-Astar*(u+cross(w,A*hr));

== matlab function Aufiero_slew_pointing/RW  CONTROL/RW REAL CONTROL/4 Reaction Wheels (2) ==
  data: w input; hr input; ureal output; hrdot input
function ureal = RW2(w,hr,hrdot)

A=[1 0 0 1/sqrt(3)
    0 1 0 1/sqrt(3)
    0 0 1 1/sqrt(3)];

ureal=-A*hrdot+cross(A*hr,w);

== matlab function Aufiero_slew_pointing/Disturbances/SRP/orbit dynamics ==
  data: x input; dy output; mp input
function dy=dynamics(x,mp)

% dynamics.m - It transform the second order differential equation of the
% equation of motion of an object that is orbiting around a planet in a
% first order system which is the form needed to use "ode45".
% a(t)=-(mu/r^3)x(t)
%
% PROTOTYPE:
%   dy = dynamics(t,x,mu)
%
% INPUT:
%   t       time instant
%   x[6]    position and velocity components
%   mu[1]   gravity constant of the considered planet (Km^3/s^2)
%
% OUTPUT:
%   dy[6]   Returns a 6 components row vector of the generalized components 
%           that I used to build up a first order system from a second 
%           order ODE
%
% CONTRIBUTORS
%
%   Alessio Cortese
%   Marco Mangialardo
%
%--------------------------------------------------------------------------
mu = mp*6.67e-11;
r=norm(x(1:3));
b=-mu/r^3;

dy=zeros(6,1);

dy(1)=x(4);
dy(2)=x(5);
dy(3)=x(6);
dy(4)=b*x(1);
dy(5)=b*x(2);
dy(6)=b*x(3);


return

== matlab function Aufiero_slew_pointing/pointing_error/ Pointing Angle Accuracy ==
  data: A_BN input; alfa_pointing_deg output; A_LN input
function alfa_pointing_deg = paa(A_BN,A_LN)

u = [1 0 0] * A_BN;
v = [1 0 0] * A_LN;

CosTheta = dot(u,v)/(norm(u)*norm(v));
alfa_pointing_deg = acosd(CosTheta);

end

== matlab function Aufiero_slew_pointing/Disturbances/SRP/A_LN ==
  data: r input; v input; A_LN output; check output
function [A_LN,check]  = ellipse_center_point(r,v)


    r1 = r./norm(r);
    
    r3 = cross(r1,v)./norm(cross(r1,v));
    
    r2 = cross(r3,r1);
    
    A_LN = [r1' ; r2' ; r3'];
    
    check = trace(A_LN'* A_LN - eye(3));
    
    
end

== matlab function Aufiero_slew_pointing/ATTITUDE DETERMINATION/Determination algorithm /Static determination/attitude determination ==
  data: h_inertial input; A_B_N output; h_measured input; B_inertial input; B_measured input
function A_B_N = ATTDET(h_inertial,h_measured,B_inertial,B_measured)

% normalization
h_inertial = h_inertial./norm(h_inertial);
h_measured = h_measured./norm(h_measured);
B_inertial = B_inertial./norm(B_inertial);
B_measured = B_measured./norm(B_measured);
        
        
% 1 = TRIAD, 2 = q method, 3 = QUEST, 4 = Single Value Decomposition
det=1;
switch det
    case 1
        
        % TRIAD
               
        % reference system based on model
        V_model = zeros(3,3);
        V_model(:,1) = h_inertial;
        V_model(:,2) = cross(h_inertial,B_inertial)./norm(cross(h_inertial,B_inertial));
        V_model(:,3) = cross(h_inertial,V_model(:,2))./norm(cross(h_inertial,V_model(:,2)));
        
        % reference system based on sensors
        V_sensor = zeros(3,3);
        V_sensor(:,1) = h_measured;
        V_sensor(:,2) = cross(h_measured,B_measured)./norm(cross(h_measured,B_measured));
        V_sensor(:,3) = cross(h_measured,V_sensor(:,2))./norm(cross(h_measured,V_sensor(:,2)));
        
        % kinematics matrix
        A_B_N = V_sensor*V_model';
        
    case 2
        
        % q method
        amag=0.2/(10+0.2);
        aeh=10/(10+0.2);
        alpha=amag+aeh; %must be 1
        
        B=amag*B_measured*B_inertial'+aeh*h_measured*h_inertial';
        
        S=B'+B;
        Z=[B(2,3)-B(3,2)
            B(3,1)-B(1,3)
            B(1,2)-B(2,1)];
        sigma=trace(B);
        I=eye(3);
        K=[S-sigma*I Z
            Z' sigma];
        
        [eigvec,eigval]=eig(K);
        q1=eigvec(1,4);
        q2=eigvec(2,4);
        q3=eigvec(3,4);
        q4=eigvec(4,4);
        
        A_B_N=[q1^2-q2^2-q3^2+q4^2 2*(q1*q2+q3*q4) 2*(q1*q3-q2*q4)
            2*(q1*q2-q3*q4) -q1^2+q2^2-q3^2+q4^2 2*(q2*q3+q1*q4)
            2*(q1*q3+q2*q4) 2*(q2*q3-q1*q4) -q1^2-q2^2+q3^2+q4^2];
        
    case 3
        
        % QUEST
        amag=0.2/(10+0.2);
        aeh=10/(10+0.2);
        alpha=amag+aeh; %must be 1
        
        B=amag*B_measured*B_inertial'+aeh*h_measured*h_inertial';
        
        S=B'+B;
        Z=[B(2,3)-B(3,2)
            B(3,1)-B(1,3)
            B(1,2)-B(2,1)];
        sigma=trace(B);
        I=eye(3);
        
        g=linsolve(S-(sigma+1)*I,-Z);
        
        A_B_N=(1/(1+g(1)^2+g(2)^2+g(3)^2))*[1+g(1)^2-g(2)^2-g(3)^2 2*(g(1)*g(2)+g(3)) 2*(g(1)*g(3)-g(2))
            2*(g(1)*g(2)-g(3)) 1-g(1)^2+g(2)^2-g(3)^2 2*(g(2)*g(3)+g(1))
            2*(g(1)*g(3)+g(2)) 2*(g(2)*g(3)-g(1)) 1-g(1)^2-g(2)^2+g(3)^2];
        
    case 4
        
        % SVD
        amag=0.2/(10+0.2);
        aeh=10/(10+0.2);
        alpha=amag+aeh; %must be 1
        
        B=amag*B_measured*B_inertial'+aeh*h_measured*h_inertial';
        
        [U,S,V]=svd(B);
        M=[1 0 0
            0 1 0
            0 0 det(U)*det(V)];
        
        A_B_N=U*M*V';
        
end

== matlab function Aufiero_slew_pointing/Reference Attitude LEO orbit/Orbital dynamics ==
  data: x0 input; x_dot output
function x_dot  = twobodyproblem(x0)

mu = 398600;

% INPUT: STATE VECTOR

r = x0(1:3);  %[1x3] position
r_dot = x0(4:6);  %[1x3] velocity


% EQUIVALENT 1st ORDER SYSTEM

p_dot = r_dot'; % derivative of the position
v_dot = ((-mu/norm(r)^3).*r)'; % derivative of the velocity

% OUTPUT: DERIVATIVE OF THE STATE VECTOR

x_dot = [p_dot v_dot]';

end

== matlab function Aufiero_slew_pointing/Reference Attitude LEO orbit/State vector from Keplerian orbital elements ==
  data: OE input; r0 output; v0 output
function [r0,v0] = sv_from_oe (OE)
% This function computes the state vector (r,v) from the classical 
% orbital elements
%
% PROTOTYPE
%   [r,v] = sv_from_oe (OE, mu)
%
% INPUT
%
% OE        orbital elements [a e i W w TA]                             [1x6]       
% mu        gravitational parameter             [km^3/s^2]
%
% OUTPUT
% r         position vector in ECI frame        [km]                    [1x3]
% v         velocity vector in ECI frame        [km/s]                  [1x3]
%
%   Verified by Daniele Leuteri Costanzo

mu = 398600;
% KEPLERIAN ORBITAL ELEMENTS
a = OE(1);
e = OE(2);
i = OE(3);
W = OE(4);
w = OE(5);
TA = OE(6);

% Semi latus rectum
p = a*(1 - norm(e)^2);

% Position and velocity in the perifocal frame

R = p/(1 + norm(e)*cos(TA));
rp = [R*cos(TA);R*sin(TA);0];
vp = [-sqrt(mu/p)*sin(TA); sqrt(mu/p)*(norm(e) + cos(TA)); 0];

% Rotation matrices
% R3_w - Rotation matrix about the z-axis through the angle w
% R1_i - Rotation matrix about the x-axis through the angle i
% R3_W - Rotation matrix about the z-axis through the angle W

R3_W = [ cos(W) sin(W) 0
        -sin(W) cos(W) 0
          0      0     1];
        
R1_i = [ 1     0       0
         0  cos(i) sin(i)
         0 -sin(i) cos(i)];
        
R3_w = [ cos(w) sin(w)   0
        -sin(w) cos(w)   0
            0       0    1];
       
% R_tot - Overall rotation from perifocal to geocentric equatorial frame
R_tot = R3_W' * R1_i' * R3_w';

% Position and velocity vectors expressed in the geocentric equatorial
% frame
r0 = R_tot*rp;
v0 = R_tot*vp;


end

== matlab function Aufiero_slew_pointing/Reference Attitude LEO orbit/LVLH frame ==
  data: r input; A_LN output; pointing_vector output; v input; check output
function [A_LN, pointing_vector, check]  = frame_tracking (r,v)
% Developing orthonormal frame to track
% r1 is the pointing vector (Earth pointing)

    r1 = r./norm(r);
    
    r3 = cross(r1,v)./norm(cross(r1,v));
    
    r2 = cross(r3,r1);
    
    pointing_vector = r1;
    
    A_LN = [r1' ; r2' ; r3'];
    
    check = trace(A_LN'*A_LN - eye(3));
  
end

== matlab function Aufiero_slew_pointing/Disturbances/SRP/SRP ==
  data: SB input; T_SRP output; dim input
function T_SRP = srp(SB, dim)

% Data
rho_d = 0.1;
rho_s = 0.5;

% Normals
n_1 = [1 0 0];
n_2 = [0 1 0];
n_3 = [0 0 1];
n_4 = [-1 0 0];
n_5 = [0 -1 0];
n_6 = [0 0 -1];

% 6U Cubesat sizes

w = dim(1); 
l = dim(2); 
h = dim(3); 

% Sections 
A_i_1 = w*l;
A_i_2 = w*h;
A_i_3 = l*h;
A_i_4 = A_i_1;
A_i_5 = A_i_2;
A_i_6 = A_i_3;

% Distance between the center of pressure and the center of mass

r_1 = [h/2 0.1 0.1];
r_2 = [0.2 l/2 0.2];
r_3 = [0.4 0.4 w/2];
r_4 = [-h/2 0.1 0.1];
r_5 = [0.2 -l/2 0.2];
r_6 = [0.4 0.4 -w/2];

% Compute Solar Radiation Pressure
% Data taken from Fundamentals of Spacecraft Attitude Determination and Control
solar_flux = 1362;        % W/m^2
c = 299792458;            % m/s
P = solar_flux/c;         % Pa

SB = SB';
   
    % Torque due to SRP, computed only on exposed surfaces.
    if dot(SB,n_1) >= 0
        F_srp_1 = P*A_i_1*dot(SB,n_1) * ((1-rho_s)*SB + (2*rho_s*dot(SB,n_1)+2/3*rho_d)*n_1);
        T_srp_1 = cross(r_1,F_srp_1);
    else
        T_srp_1 = [0 0 0];
    end
    
    if dot(SB,n_2) >= 0
        F_srp_2 = P*A_i_2*dot(SB,n_2) * ((1-rho_s)*SB + (2*rho_s*dot(SB,n_2)+2/3*rho_d)*n_2);
        T_srp_2 = cross(r_2,F_srp_2);
    else
        T_srp_2 = [0 0 0];
    end
    
    if dot(SB,n_3) >= 0
        F_srp_3 = P*A_i_3*dot(SB,n_3) * ((1-rho_s)*SB + (2*rho_s*dot(SB,n_3)+2/3*rho_d)*n_3);
        T_srp_3 = cross(r_3,F_srp_3);
    else
        T_srp_3 = [0 0 0];
    end
    
    if dot(SB,n_4) >= 0
        F_srp_4 = P*A_i_4*dot(SB,n_4) * ((1-rho_s)*SB + (2*rho_s*dot(SB,n_4)+2/3*rho_d)*n_4);
        T_srp_4 = cross(r_4,F_srp_4);
    else
        T_srp_4 = [0 0 0];
    end
    
    if dot(SB,n_5) >= 0
        F_srp_5 = P*A_i_5*dot(SB,n_5) * ((1-rho_s)*SB + (2*rho_s*dot(SB,n_5)+2/3*rho_d)*n_5);
        T_srp_5 = cross(r_5,F_srp_5);
    else
        T_srp_5 = [0 0 0];
    end
    
    if dot(SB,n_6) >= 0
        F_srp_6 = P*A_i_6*dot(SB,n_6) * ((1-rho_s)*SB + (2*rho_s*dot(SB,n_6)+2/3*rho_d)*n_6);
        T_aero_6 = cross(r_6,F_srp_6);
    else
        T_aero_6 = [0 0 0];
    end
    
    T_SRP = T_srp_1 + T_srp_2 + T_srp_3 + T_srp_4 + T_srp_5 + T_srp_5 + T_aero_6;
end

== matlab function Aufiero_slew_pointing/Reference Attitude LEO orbit/A_LN trace check/Orthonormality check ==
  data: A_LN input; t output
function t = trace(A_LN)
% Checking orthonormality

tr_ALN = trace(eye(3)- A_LN.' * A_LN);

t = tr_ALN;

== matlab function Aufiero_slew_pointing/Disturbances/Gravity gradient/Gravity Gradient ==
  data: I input; T_GG output; A_LN input; A_BN input; r input
function T_GG = dist_gravity_gradient(I,A_LN, A_BN, r)
 
    mu = 398600; 
    R_earth = 6378;
    n = sqrt(mu/R_earth);
    
    
    A_BL = A_BN * A_LN';
    
    
    c = A_BL*[1;0;0];
    
    T_GG = zeros(1,3);
    
    T_GG(1) = (3 * n^2) * (I(3)-I(2)) * c(3) * c(2)/(I(1)*norm(r)^3);
    T_GG(2) = (3 * n^2) * (I(1)-I(3)) * c(1) * c(3)/(I(2)*norm(r)^3);
    T_GG(3) = (3 * n^2) * (I(2)-I(1)) * c(2) * c(1)/(I(3)*norm(r)^3);
    
end

== matlab function Aufiero_slew_pointing/Disturbances/SRP/Orbital Parameter are refeered to Earth's orbit around the Sun.    ==
  data: a input; e input; r0 output; i input; v0 output; Omega input; omega input; teta input; mp input
function [r0,v0]=kep2car(a,e,i,Omega,omega,teta,mp)

% kep2car.m - the function computes cartesian coordinates
% (position vector and velocity) starting from keplerian
% parameters
%
%
% PROTOTYPE:
%   [r,v]=kep2car(a,e,i,Omega,omega,teta,mu)
%
% INPUT:
%   a[1]        semi major axis of the orbit (m)
%   e[1]        eccentricity of the orbit
%   i[1]        inclination of the orbit wrt equatorial plane (rad)
%   Omega[1]    right asention of the ascending node (rad)
%   omega[1]    pericenter anomaly (rad)
%   teta[1]     true anomaly of the spacecraft wrt its pericenter (rad)
%
% OUTPUT:
%   r[3]    vector containing the spacecraft position (x,y,z) (m)
%   v[3]    vector containing the spacecraft velocity components (m/s)
%   mp[1]   mass of the planet (kg)
%
% CONTRIBUTORS
%
%   Alessio Cortese
%   Marco Mangialardo
%
%--------------------------------------------------------------------------

mu = mp*6.67e-11;

p=a*(1-e^2);

rho=p/(1+e*cos(teta));
r_pf=[rho*cos(teta); rho*sin(teta); 0];

v_pf=[-sqrt(mu/p)*sin(teta); sqrt(mu/p)*(e+cos(teta)); 0];

Omega_mat=[ cos(Omega) sin(Omega)           0;
           -sin(Omega) cos(Omega)           0;
                    0          0            1];   %rotaz Omega intorno k_pf

i_mat=[             1          0            0;
                    0      cos(i)      sin(i);
                    0     -sin(i)      cos(i)];
                
omega_mat=[ cos(omega) sin(omega)           0;
           -sin(omega) cos(omega)           0;
                    0          0            1];
                
 Tge_pf=(omega_mat)*(i_mat)*(Omega_mat); %rotaz geoc a perifoc
 
 Tpf_ge=Tge_pf';
 
 r0=Tpf_ge*r_pf;
 v0=Tpf_ge*v_pf;
end
